simulink library "momentum_dump_lib_test"  (R2016b)
settings: Solver=VariableStepAuto  StartTime=0.0  StopTime=10.0  RelTol=1e-3
values from neighbouring files (symbols this model uses):
  fsw_params = init_fsw_params()    [momentum_unload_test_init.m]
settings Model: Creator=unsik  LastModifiedBy=evich

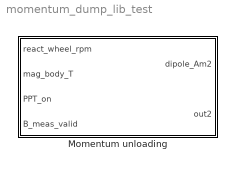
== system momentum_dump_lib_test ==
  Momentum unloading : Subsystem

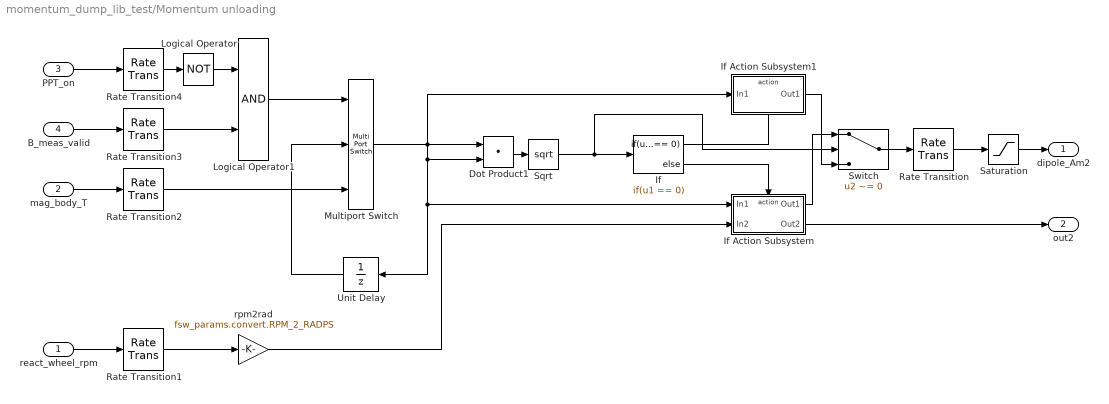
== system momentum_dump_lib_test/Momentum unloading ==
  react_wheel_rpm : Inport
  mag_body_T : Inport  Port=2
  PPT_on : Inport  Port=3
  B_meas_valid : Inport  Port=4
  Dot Product1 : DotProduct  InputSameDT=on  OutDataTypeStr=Inherit: Inherit via internal rule
  If : If  IfExpression=u1 == 0
  If Action Subsystem : Subsystem  TreatAsAtomicUnit=on
  If Action Subsystem1 : Subsystem  TreatAsAtomicUnit=on
  Logical Operator : Logic  Operator=NOT  AllPortsSameDT=off  OutDataTypeStr=boolean
  Logical Operator1 : Logic  AllPortsSameDT=off  OutDataTypeStr=boolean
  Multiport Switch : MultiPortSwitch  DataPortOrder=Zero-based contiguous  Inputs=2
  Rate Transition : RateTransition  X0=fsw_params.control.p_dump.ic.rt_dipole_Am2
  Rate Transition1 : RateTransition  X0=fsw_params.control.p_dump.ic.rt_w_body_radps  OutPortSampleTime=fsw_params.control.p_dump.sample_time_s
  Rate Transition2 : RateTransition  X0=fsw_params.control.p_dump.ic.rt_mag_body_T  OutPortSampleTime=fsw_params.control.p_dump.sample_time_s
  Rate Transition3 : RateTransition  X0=fsw_params.control.p_dump.ic.rt_B_meas_valid  OutPortSampleTime=fsw_params.control.p_dump.sample_time_s
  Rate Transition4 : RateTransition  X0=fsw_params.control.p_dump.ic.rt_PPT_on  OutPortSampleTime=fsw_params.control.p_dump.sample_time_s
  Saturation : Saturate
  Sqrt : Sqrt  SaturateOnIntegerOverflow=on
  Switch : Switch  Criteria=u2 ~= 0
  Unit Delay : UnitDelay  InitialCondition=fsw_params.control.p_dump.ic.delay  SampleTime=-1
  rpm2rad : Gain  Gain=fsw_params.convert.RPM_2_RADPS
  dipole_Am2 : Outport
  out2 : Outport  Port=2
  wires:
  Logical Operator1/1 -> Multiport Switch/1
  Logical Operator/1 -> Logical Operator1/1
  Rate Transition3/1 -> Logical Operator1/2
  Rate Transition4/1 -> Logical Operator/1
  Rate Transition2/1 -> Multiport Switch/3
  Unit Delay/1 -> Multiport Switch/2
  PPT_on/1 -> Rate Transition4/1
  B_meas_valid/1 -> Rate Transition3/1
  mag_body_T/1 -> Rate Transition2/1
  Rate Transition/1 -> Saturation/1
  react_wheel_rpm/1 -> Rate Transition1/1
  Multiport Switch/1 -> If Action Subsystem1/1(In1), Dot Product1/1, Dot Product1/2, If Action Subsystem/1(In1), Unit Delay/1
  Dot Product1/1 -> Sqrt/1
  Sqrt/1 -> Switch/2, If/1
  If/2 -> If Action Subsystem/Action
  If/1 -> If Action Subsystem1/Action
  If Action Subsystem1/1(Out1) -> Switch/3
  If Action Subsystem/1(Out1) -> Switch/1
  Rate Transition1/1 -> rpm2rad/1
  rpm2rad/1 -> If Action Subsystem/2(In2)
  If Action Subsystem/2(Out2) -> out2/1
  Switch/1 -> Rate Transition/1
  Saturation/1 -> dipole_Am2/1

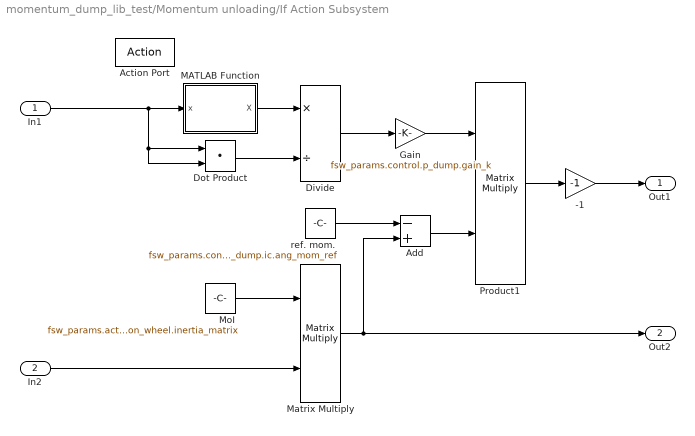
== system momentum_dump_lib_test/Momentum unloading/If Action Subsystem ==
  In1 : Inport
  In2 : Inport  Port=2
  Action Port : ActionPort  ActionType=else
  -1 : Gain  Gain=-1
  Add : Sum  Inputs=-+
  Divide : Product  Inputs=*/
  Dot Product : DotProduct  InputSameDT=on  OutDataTypeStr=Inherit: Inherit via internal rule
  Gain : Gain  Gain=fsw_params.control.p_dump.gain_k
  MATLAB Function : MATLAB Function  TreatAsAtomicUnit=on
  Matrix Multiply : Product  Inputs=**  Multiplication=Matrix(*)
  MoI : Constant  Value=fsw_params.actuators.reaction_wheel.inertia_matrix
  Product1 : Product  Inputs=**  Multiplication=Matrix(*)
  ref. mom. : Constant  Value=fsw_params.control.p_dump.ic.ang_mom_ref
  Out1 : Outport
  Out2 : Outport  Port=2
  wires:
  Divide/1 -> Gain/1
  Dot Product/1 -> Divide/2
  ref. mom./1 -> Add/1
  Matrix Multiply/1 -> Out2/1, Add/2
  MATLAB Function/1(X) -> Divide/1
  MoI/1 -> Matrix Multiply/1
  In1/1 -> Dot Product/2, Dot Product/1, MATLAB Function/1(x)
  In2/1 -> Matrix Multiply/2
  Product1/1 -> -1/1
  Add/1 -> Product1/2
  -1/1 -> Out1/1
  Gain/1 -> Product1/1

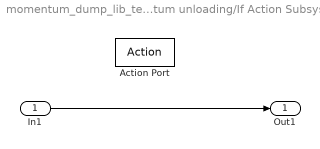
== system momentum_dump_lib_test/Momentum unloading/If Action Subsystem1 ==
  In1 : Inport
  Action Port : ActionPort  ActionType=then
  Out1 : Outport
  wires:
  In1/1 -> Out1/1

== matlab function momentum_dump_lib_test/Momentum unloading/If Action Subsystem/MATLAB Function ==
  data: x input; X output
function X   = skew( x )
% UW HuskySat-1, ADCS Subsystem
% Last Update: E. Hansen 12.8.2017

%Transforms a vector into a skew symmetric matrix (Levi-Civita)
%--------------------------------------------------------------------------

X = [0 -x(3) x(2);x(3) 0 -x(1);-x(2) x(1) 0];
